simulink model "sampleModel1759"  (R2023a)
settings: Solver=VariableStepAuto  StartTime=0.0  StopTime=10.0  RelTol=1e-3
libraries: hdlsllib x6, simulink x2
settings Model: Creator=user1  LastModifiedBy=user1

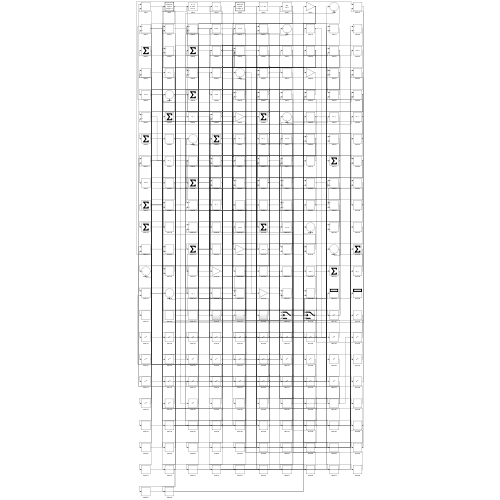
[thumbnail: Simulink's stored preview of the top-level diagram]
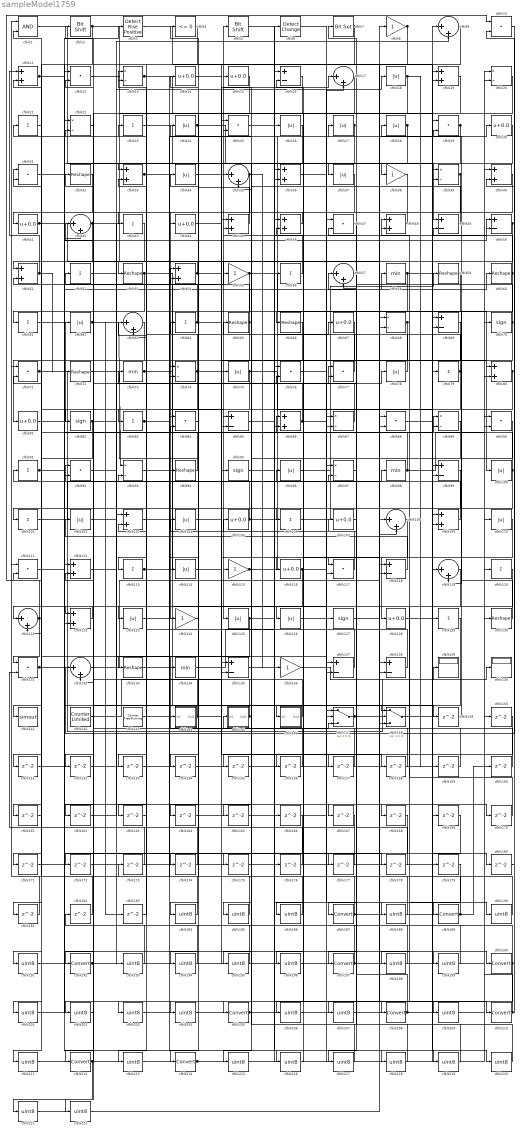
== system sampleModel1759 ==
  cfblk1 : Logic  AllPortsSameDT=off  OutDataTypeStr=boolean
  cfblk{10,12,25,29,31,47,71,76..77,84,88,90,92,111,117,131} (16 alike) : DotProduct  OutDataTypeStr=Inherit: Inherit via internal rule
  cfblk{18,24,26..28,34,37,62,75,78,96,100,102,104,110,114,123,125..126} (19 alike) : Abs  SaturateOnIntegerOverflow=off
  cfblk{21,23,43,52,56,61,64,79,83,91,101,106,113,120,129} (15 alike) : Sum  Inputs=+
  cfblk{11,19,33,36,40,45..46,48,51,54,80,86,103,109,112,122} (16 alike) : Sum
  cfblk{14..15,30,41,44,67,81,105,107,116,128} (11 alike) : Bias  Bias=0.0  SaturateOnIntegerOverflow=off
  cfblk{9,17,35,42,57,63,108,119,121,132} (10 alike) : Sum  Inputs=|++
  cfblk{8,38,55,115,124,136} (6 alike) : Gain
  cfblk{16,49..50,69,85,99,118,135,137..138} (10 alike) : Sum  Inputs=+-
  cfblk{70,82,95,127} (4 alike) : Signum
  cfblk{13,20,22,39,68,74,87,89,93,97} (10 alike) : Product  Inputs=*/  RndMeth=Zero  SaturateOnIntegerOverflow=on
  cfblk{32,53,59..60,65..66,72,94,130,133} (10 alike) : Reshape
  cfblk{58,73,98,134} (4 alike) : MinMax
  cfblk139 : Display
  cfblk140 : Display
  cfblk141 : ToWorkspace  VariableName=simout  SaveFormat=Timeseries  SampleTime=-1
  cfblk142 : hdlsllib/Sources/Counter Limited  uplimit=7  tsamp=-1
  cfblk143 : hdlsllib/Sources/Counter Free-Running  NumBits=16  tsamp=-1
  cfblk144 : Subsystem
      settings: LibrarySourceBlock=|
      | hdlsllib/Ports &
      | Subsystems/Subsystem
  cfblk145 : Subsystem
      settings: LibrarySourceBlock=|
      | hdlsllib/Ports &
      | Subsystems/Subsystem
  cfblk146 : Subsystem
      settings: LibrarySourceBlock=|
      | hdlsllib/Ports &
      | Subsystems/Subsystem
  cfblk147 : Switch  SaturateOnIntegerOverflow=off  InputSameDT=off
  cfblk148 : Switch  SaturateOnIntegerOverflow=off  InputSameDT=off
  cfblk{149..183} (35 alike) : Delay  SampleTime=1
  cfblk{184..186,188,190..191,193..196,198..199,201..204,206..207,209,211,213,215..222} (29 alike) : DataTypeConversion  OutDataTypeStr=uint8  SaturateOnIntegerOverflow=off  RndMeth=Floor
  cfblk{187,189,192,197,200,205,208,210,212,214} (10 alike) : DataTypeConversion  SaturateOnIntegerOverflow=off  RndMeth=Floor
  cfblk2 : hdlsllib/Logic and Bit Operations/Bit Shift  mode=Shift Left Logical  N=0
  cfblk3 : hdlsllib/Logic and Bit Operations/Detect Rise Positive  vinit=0  OutDataTypeStr=boolean
  cfblk4 : hdlsllib/Logic and Bit Operations/Compare To Zero  relop=<=  OutDataTypeStr=boolean
  cfblk5 : hdlsllib/Logic and Bit Operations/Bit Shift  mode=Shift Left Logical  N=0
  cfblk6 : simulink/Logic and Bit Operations/Detect Change  vinit=0  OutDataTypeStr=boolean
      settings: LibrarySourceBlock=|
      | hdlsllib/Logic and Bit
      | Operations/Detect
      | Change
  cfblk7 : simulink/Logic and Bit Operations/Bit Set  iBit=0
      settings: LibrarySourceBlock=|
      | hdlsllib/Logic and Bit
      | Operations/Bit Set
  wires:
  cfblk53/1 -> cfblk146/1(In1), cfblk191/1
  cfblk107/1 -> cfblk187/1
  cfblk137/1 -> cfblk34/1
  cfblk133/1 -> cfblk145/1(In1)
  cfblk43/1 -> cfblk53/1
  cfblk148/1 -> cfblk89/1
  cfblk1/1 -> cfblk49/1
  cfblk71/1 -> cfblk139/1, cfblk3/1
  cfblk37/1 -> cfblk124/1
  cfblk47/1 -> cfblk197/1
  cfblk130/1 -> cfblk92/1
  cfblk16/1 -> cfblk214/1
  cfblk48/1 -> cfblk41/1
  cfblk2/1 -> cfblk39/1, cfblk211/1
  cfblk106/1 -> cfblk59/1
  cfblk113/1 -> cfblk77/1, cfblk60/1, cfblk96/1
  cfblk34/1 -> cfblk5/1
  cfblk7/1 -> cfblk92/2, cfblk86/2
  cfblk19/1 -> cfblk126/1
  cfblk23/1 -> cfblk138/1
  cfblk60/1 -> cfblk28/1, cfblk119/2
  cfblk68/1 -> cfblk153/1, cfblk154/1
  cfblk51/1 -> cfblk11/1, cfblk72/1
  cfblk50/1 -> cfblk125/1, cfblk172/1
  cfblk134/1 -> cfblk6/1
  cfblk116/1 -> cfblk17/2, cfblk162/1
  cfblk10/1 -> cfblk132/1
  cfblk78/1 -> cfblk52/1
  cfblk59/1 -> cfblk115/1
  cfblk65/1 -> cfblk31/1, cfblk74/2
  cfblk102/1 -> cfblk78/1
  cfblk100/1 -> cfblk101/1, cfblk71/2
  cfblk73/1 -> cfblk137/1, cfblk13/1
  cfblk67/1 -> cfblk132/2
  cfblk87/1 -> cfblk2/1
  cfblk39/1 -> cfblk155/1, cfblk186/1
  cfblk105/1 -> cfblk30/1, cfblk13/2
  cfblk22/1 -> cfblk192/1
  cfblk49/1 -> cfblk24/1
  cfblk8/1 -> cfblk113/1, cfblk135/2, cfblk148/2
  cfblk147/1 -> cfblk69/2, cfblk50/2
  cfblk70/1 -> cfblk7/1, cfblk207/1
  cfblk64/1 -> cfblk54/1, cfblk17/1
  cfblk96/1 -> cfblk68/1
  cfblk75/1 -> cfblk89/2, cfblk85/2
  cfblk13/1 -> cfblk135/1, cfblk175/1
  cfblk12/1 -> cfblk108/2
  cfblk82/1 -> cfblk9/2, cfblk151/1
  cfblk81/1 -> cfblk62/1
  cfblk62/1 -> cfblk93/1, cfblk183/1
  cfblk127/1 -> cfblk210/1
  cfblk123/1 -> cfblk27/1
  cfblk115/1 -> cfblk67/1, cfblk177/1
  cfblk121/1 -> cfblk10/1, cfblk131/1
  cfblk122/1 -> cfblk121/1
  cfblk58/1 -> cfblk66/1, cfblk180/1
  cfblk28/1 -> cfblk164/1, cfblk165/1, cfblk206/1
  cfblk136/1 -> cfblk140/1
  cfblk55/1 -> cfblk100/1, cfblk133/1
  cfblk29/1 -> cfblk33/1, cfblk74/1
  cfblk72/1 -> cfblk144/1(In1)
  cfblk41/1 -> cfblk95/1, cfblk170/1
  cfblk146/1(Out1) -> cfblk23/1
  cfblk74/1 -> cfblk21/1, cfblk80/1, cfblk181/1
  cfblk110/1 -> cfblk128/1
  cfblk94/1 -> cfblk32/1
  cfblk101/1 -> cfblk56/1
  cfblk104/1 -> cfblk116/1
  cfblk42/1 -> cfblk87/2, cfblk121/2, cfblk137/2
  cfblk18/1 -> cfblk94/1, cfblk159/1
  cfblk54/1 -> cfblk51/1, cfblk149/1
  cfblk93/1 -> cfblk35/1
  cfblk145/1(Out1) -> cfblk91/1, cfblk25/2
  cfblk112/1 -> cfblk200/1
  cfblk45/1 -> cfblk14/1
  cfblk132/1 -> cfblk68/2
  cfblk35/1 -> cfblk82/1, cfblk136/1
  cfblk27/1 -> cfblk122/1, cfblk122/2
  cfblk142/1 -> cfblk45/1
  cfblk86/1 -> cfblk73/1, cfblk190/1
  cfblk80/1 -> cfblk83/1, cfblk134/1
  cfblk76/1 -> cfblk97/1
  cfblk11/1 -> cfblk148/3, cfblk199/1
  cfblk117/1 -> cfblk64/1
  cfblk91/1 -> cfblk86/1, cfblk58/1, cfblk178/1
  cfblk103/1 -> cfblk19/1
  cfblk111/1 -> cfblk55/1
  cfblk83/1 -> cfblk85/1, cfblk167/1
  cfblk69/1 -> cfblk114/1
  cfblk143/1 -> cfblk98/1
  cfblk63/1 -> cfblk81/1
  cfblk124/1 -> cfblk104/1
  cfblk109/1 -> cfblk63/1
  cfblk126/1 -> cfblk147/1
  cfblk120/1 -> cfblk208/1
  cfblk25/1 -> cfblk37/1
  cfblk77/1 -> cfblk15/1
  cfblk4/1 -> cfblk43/1
  cfblk138/1 -> cfblk103/2
  cfblk90/1 -> cfblk205/1
  cfblk97/1 -> cfblk117/1
  cfblk21/1 -> cfblk61/1
  cfblk36/1 -> cfblk189/1
  cfblk3/1 -> cfblk79/1
  cfblk40/1 -> cfblk109/2
  cfblk144/1(Out1) -> cfblk93/2, cfblk147/3
  cfblk99/1 -> cfblk123/1
  cfblk24/1 -> cfblk38/1, cfblk117/2
  cfblk33/1 -> cfblk213/1, cfblk216/1
  cfblk118/1 -> cfblk102/1
  cfblk92/1 -> cfblk18/1
  cfblk114/1 -> cfblk29/2
  cfblk56/1 -> cfblk45/2
  cfblk32/1 -> cfblk141/1
  cfblk46/1 -> cfblk44/1
  cfblk131/1 -> cfblk148/1, cfblk50/1
  cfblk79/1 -> cfblk46/2, cfblk106/1
  cfblk9/1 -> cfblk138/2
  cfblk98/1 -> cfblk20/2, cfblk4/1
  cfblk31/1 -> cfblk42/2
  cfblk125/1 -> cfblk48/1, cfblk171/1
  cfblk44/1 -> cfblk118/2
  cfblk129/1 -> cfblk212/1
  cfblk149/1 -> cfblk49/2
  cfblk151/1 -> cfblk54/2
  cfblk20/1 -> cfblk152/1
  cfblk152/1 -> cfblk29/1
  cfblk153/1 -> cfblk69/1
  cfblk154/1 -> cfblk19/2
  cfblk155/1 -> cfblk109/1
  cfblk14/1 -> cfblk156/1
  cfblk156/1 -> cfblk42/1
  cfblk89/1 -> cfblk157/1
  cfblk157/1 -> cfblk76/2
  cfblk85/1 -> cfblk158/1
  cfblk158/1 -> cfblk35/2
  cfblk159/1 -> cfblk118/1
  cfblk160/1 -> cfblk46/1
  cfblk119/1 -> cfblk161/1
  cfblk161/1 -> cfblk11/2
  cfblk162/1 -> cfblk103/1
  cfblk15/1 -> cfblk163/1
  cfblk163/1 -> cfblk33/2
  cfblk164/1 -> cfblk87/1
  cfblk165/1 -> cfblk147/2
  cfblk167/1 -> cfblk131/2
  cfblk6/1 -> cfblk168/1
  cfblk170/1 -> cfblk48/2
  cfblk171/1 -> cfblk39/2
  cfblk172/1 -> cfblk99/2
  cfblk173/1 -> cfblk111/2
  cfblk30/1 -> cfblk174/1
  cfblk174/1 -> cfblk31/2
  cfblk175/1 -> cfblk9/1
  cfblk176/1 -> cfblk71/1
  cfblk177/1 -> cfblk51/2
  cfblk178/1 -> cfblk97/2
  cfblk128/1 -> cfblk179/1
  cfblk180/1 -> cfblk40/2
  cfblk181/1 -> cfblk1/1
  cfblk182/1 -> cfblk1/2
  cfblk183/1 -> cfblk63/2
  cfblk84/1 -> cfblk184/1
  cfblk184/1 -> cfblk111/1
  cfblk168/1 -> cfblk185/1
  cfblk185/1 -> cfblk84/1
  cfblk186/1 -> cfblk84/2
  cfblk187/1 -> cfblk25/1, cfblk119/1
  cfblk95/1 -> cfblk188/1
  cfblk188/1 -> cfblk107/1
  cfblk189/1 -> cfblk173/1, cfblk160/1, cfblk99/1
  cfblk190/1 -> cfblk36/1
  cfblk191/1 -> cfblk36/2
  cfblk192/1 -> cfblk176/1, cfblk70/1, cfblk75/1
  cfblk52/1 -> cfblk193/1
  cfblk193/1 -> cfblk22/1
  cfblk166/1 -> cfblk194/1
  cfblk194/1 -> cfblk22/2
  cfblk150/1 -> cfblk195/1
  cfblk195/1 -> cfblk12/2
  cfblk108/1 -> cfblk196/1
  cfblk196/1 -> cfblk150/1
  cfblk197/1 -> cfblk40/1, cfblk12/1
  cfblk179/1 -> cfblk198/1
  cfblk198/1 -> cfblk47/1
  cfblk199/1 -> cfblk47/2
  cfblk200/1 -> cfblk76/1, cfblk222/1
  cfblk38/1 -> cfblk201/1
  cfblk201/1 -> cfblk112/1
  cfblk169/1 -> cfblk202/1
  cfblk202/1 -> cfblk112/2
  cfblk26/1 -> cfblk203/1
  cfblk203/1 -> cfblk8/1
  cfblk17/1 -> cfblk204/1
  cfblk204/1 -> cfblk26/1
  cfblk205/1 -> cfblk166/1, cfblk80/2
  cfblk206/1 -> cfblk90/1
  cfblk207/1 -> cfblk90/2
  cfblk208/1 -> cfblk169/1, cfblk77/2
  cfblk135/1 -> cfblk209/1
  cfblk209/1 -> cfblk120/1
  cfblk210/1 -> cfblk10/2, cfblk20/1
  cfblk211/1 -> cfblk127/1
  cfblk212/1 -> cfblk182/1, cfblk221/1
  cfblk213/1 -> cfblk129/1
  cfblk214/1 -> cfblk130/1, cfblk110/1, cfblk108/1
  cfblk66/1 -> cfblk215/1
  cfblk215/1 -> cfblk16/1
  cfblk216/1 -> cfblk16/2
  cfblk57/1 -> cfblk217/1
  cfblk217/1 -> cfblk105/1
  cfblk5/1 -> cfblk218/1
  cfblk218/1 -> cfblk57/1
  cfblk61/1 -> cfblk219/1
  cfblk219/1 -> cfblk57/2
  cfblk88/1 -> cfblk220/1
  cfblk220/1 -> cfblk65/1
  cfblk221/1 -> cfblk88/1
  cfblk222/1 -> cfblk88/2

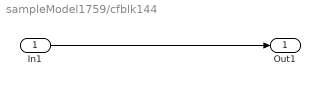
== system sampleModel1759/cfblk144 ==
  In1 : Inport
  Out1 : Outport
  wires:
  In1/1 -> Out1/1

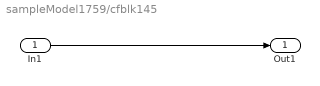
== system sampleModel1759/cfblk145 ==
  In1 : Inport
  Out1 : Outport
  wires:
  In1/1 -> Out1/1

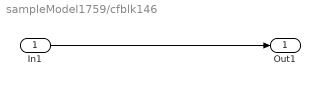
== system sampleModel1759/cfblk146 ==
  In1 : Inport
  Out1 : Outport
  wires:
  In1/1 -> Out1/1
